simulink model "fishhook_test"  (Simulink 10.1)
settings: Solver=ode45  StartTime=0  StopTime=20  FixedStep=0.002  RelTol=1e-3  AbsTol=1e-6
PreLoadFcn:
  | m=7620;
  | a=3.105;
  | b=1.385;
  | mu=0.85;
  | g=9.8;
  | k1=-220;
  | k2=-480;
libraries: simulink x2, Solver_SF x1
settings Model: Creator=bduprey  LastModifiedBy=Lenovo  ExtModeTrigMode=oneshot  ExtModeArmWhenConnect=off
settings SolverCC: AutoScaleAbsTol=off
settings DataIOCC: SignalLoggingSaveFormat=ModelDataLogs
settings OptimizationCC: BlockReduction=off  BooleanDataType=off  ExpressionDepthLimit=2147483647
settings DebuggingCC: SaveWithParameterizedLinksMsg=none  SignalResolutionControl=TryResolveAllWithWarning  MultiTaskDSMMsg=warning  MultiTaskCondExecSysMsg=none  FcnCallInpInsideContextMsg=warning  StateNameClashWarn=warning
settings HardwareCC: TargetUnknown=on
settings RTWCC: TemplateMakefile=grt_vc.tmf
settings GRTTargetCC: TargetFcnLib=ansi_tfl_tmw.mat

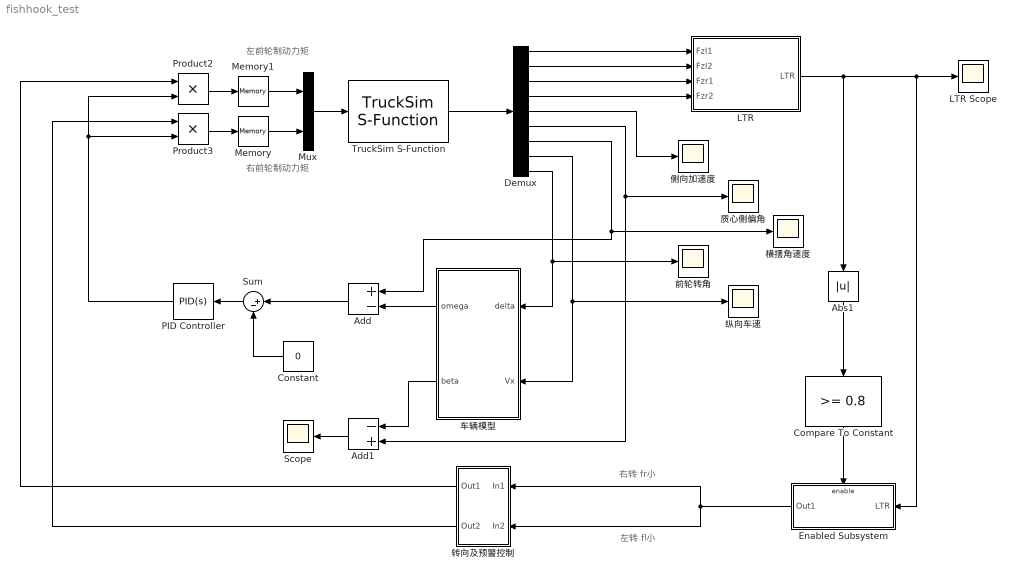
== system fishhook_test ==
  note: 左前轮制动力矩
  note: 左转 fl小
  note: 右转 fr小
  note: 右前轮制动力矩
  Abs1 : Abs
  Add : Sum  Inputs=+-
  Add1 : Sum  Inputs=-+
  Compare To Constant : simulink/Logic and Bit Operations/Compare To Constant  relop=>=  const=0.8  OutDataTypeStr=boolean
  Constant : Constant  Value=0
  Demux : Demux  Outputs=9
  Enabled Subsystem : Subsystem  TreatAsAtomicUnit=on
  LTR : Subsystem
  LTR Scope : Scope
  Memory : Memory
  Memory1 : Memory
  Mux : Mux  Inputs=2
  PID Controller : simulink/Continuous/PID Controller  Controller=PID  Form=Parallel  TimeDomain=Continuous-time  UseExternalTs=off  SampleTime=-1  IntegratorMethod=Forward Euler  FilterMethod=Forward Euler  ControllerParametersSource=internal  P=5  I=2  D=1  UseFilter=on  N=100  TunerSelectOption=Transfer Function Based (PID Tuner App)  InitialConditionSource=internal  InitialConditionForIntegrator=0  InitialConditionForFilter=0  DifferentiatorICPrevScaledInput=0  ExternalReset=none  TrackingMode=off  Kt=1  LimitOutput=off  UpperSaturationLimit=inf  LowerSaturationLimit=-inf  LinearizeAsGain=on  AntiWindupMode=none  Kb=1  POutMin=[]  POutMax=[]  IOutMin=[]  IOutMax=[]  DOutMin=[]  DOutMax=[]  NOutMin=[]  NOutMax=[]  SumOutMin=[]  SumOutMax=[]  SaturationOutMin=[]  SaturationOutMax=[]  PParamMin=[]  PParamMax=[]  IParamMin=[]  IParamMax=[]  DParamMin=[]  DParamMax=[]  NParamMin=[]  NParamMax=[]  KbParamMin=[]  KbParamMax=[]  KtParamMin=[]  KtParamMax=[]  KbOutMin=[]  KbOutMax=[]  KtOutMin=[]  KtOutMax=[]  IntegratorOutMin=[]  IntegratorOutMax=[]  FilterOutMin=[]  FilterOutMax=[]  SumI1OutMin=[]  SumI1OutMax=[]  SumI2OutMin=[]  SumI2OutMax=[]  SumI3OutMin=[]  SumI3OutMax=[]  SumI4OutMin=[]  SumI4OutMax=[]  SumDOutMin=[]  SumDOutMax=[]  DifferentiatorOutMin=[]  DifferentiatorOutMax=[]  FilterDiffOutCoefMin=[]  FilterDiffOutCoefMax=[]  ReciprocalOutMin=[]  ReciprocalOutMax=[]  SumDenOutMin=[]  SumDenOutMax=[]  SumNumOutMin=[]  SumNumOutMax=[]  DivideOutMin=[]  DivideOutMax=[]  UdiffTsProdOutMin=[]  UdiffTsProdOutMax=[]  NTsProdOutMin=[]  NTsProdOutMax=[]  UintegralTsProdOutMin=[]  UintegralTsProdOutMax=[]  UngainTsProdOutMin=[]  UngainTsProdOutMax=[]  IntegratorContinuousStateAttributes=''  IntegratorStateMustResolveToSignalObject=off  IntegratorRTWStateStorageClass=Auto  FilterContinuousStateAttributes=''  FilterStateMustResolveToSignalObject=off  FilterRTWStateStorageClass=Auto  ParallelPVariant=InternalParameters  IdealPVariant=Disabled  IVariant=InternalParameters  DVariant=InternalParameters  IntegratorVariant=Continuous  SatVariant=Disabled  AWVariant=Passthrough  PCopyVariant=Disabled  TRVariant=Disabled  FdbkBlocksVariant=Forward  IdealPFdbkVariant=Disabled  SatFdbkVariant=Disabled  DerivativeFilterVariant=ContFilter  NVariant=InternalParameters  NCopyVariant=Disabled  FilterICVariant=InternalICsFilter  IntegratorICVariant=InternalICs  ExternalResetVariant=Disabled  TRSumVariant=Passthrough  SumFdbkVariant=Disabled  SumVariant=Sum_PID  TsampFilterVariant=InternalTs  TsampNgainVariant=Passthrough  TsampIntegralVariant=Passthrough
  Product2 : Product
  Product3 : Product
  Scope : Scope
  Sum : Sum  Inputs=|+-
  TruckSim S-Function : Solver_SF/TruckSim S-Function  Priority=1  VehicleCode=i_s  SIMFILE=simfile.sim
      settings: AttributesFormatString=Vehicle Code: %<VehicleCode>
  侧向加速度 : Scope
  前轮转角 : Scope
  横摆角速度 : Scope
  纵向车速 : Scope
  质心侧偏角 : Scope
  车辆模型 : Subsystem
  转向及预警控制 : Subsystem
  wires:
  Mux/1 -> TruckSim S-Function/1
  TruckSim S-Function/1 -> Demux/1
  Demux/1 -> LTR/1(Fzl1)
  Demux/2 -> LTR/2(Fzl2)
  Demux/5 -> 侧向加速度/1
  Demux/6 -> Add1/2, 质心侧偏角/1
  Demux/7 -> Add/1, 横摆角速度/1
  LTR/1(LTR) -> Abs1/1, LTR Scope/1, Enabled Subsystem/1(LTR)
  Enabled Subsystem/1(Out1) -> 转向及预警控制/2(In2), 转向及预警控制/1(In1)
  Abs1/1 -> Compare To Constant/1
  Compare To Constant/1 -> Enabled Subsystem/Enable
  Demux/3 -> LTR/3(Fzr1)
  Demux/4 -> LTR/4(Fzr2)
  Demux/8 -> 车辆模型/2(Vx), 纵向车速/1
  Demux/9 -> 车辆模型/1(delta), 前轮转角/1
  车辆模型/1(omega) -> Add/2
  车辆模型/2(beta) -> Add1/1
  Add1/1 -> Scope/1
  Constant/1 -> Sum/2
  Add/1 -> Sum/1
  Sum/1 -> PID Controller/1
  转向及预警控制/1(Out1) -> Product2/1
  转向及预警控制/2(Out2) -> Product3/1
  Product2/1 -> Memory1/1
  Product3/1 -> Memory/1
  Memory1/1 -> Mux/1
  Memory/1 -> Mux/2
  PID Controller/1 -> Product3/2, Product2/2

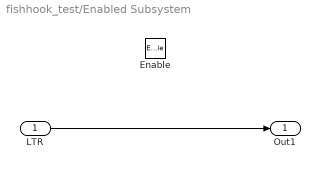
== system fishhook_test/Enabled Subsystem ==
  LTR : Inport
  Enable : EnablePort  ShowOutputPort=on
  Out1 : Outport
  wires:
  LTR/1 -> Out1/1

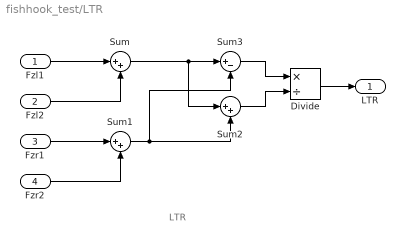
== system fishhook_test/LTR ==
  note: LTR
  Fzl1 : Inport
  Fzl2 : Inport  Port=2
  Fzr1 : Inport  Port=3
  Fzr2 : Inport  Port=4
  Divide : Product  Inputs=*/
  Sum : Sum  Inputs=|++
  Sum1 : Sum  Inputs=|++
  Sum2 : Sum  Inputs=|++
  Sum3 : Sum  Inputs=|+-
  LTR : Outport
  wires:
  Divide/1 -> LTR/1
  Sum1/1 -> Sum3/2, Sum2/2
  Fzl2/1 -> Sum/2
  Fzr1/1 -> Sum1/1
  Sum2/1 -> Divide/2
  Sum3/1 -> Divide/1
  Fzl1/1 -> Sum/1
  Fzr2/1 -> Sum1/2
  Sum/1 -> Sum2/1, Sum3/1

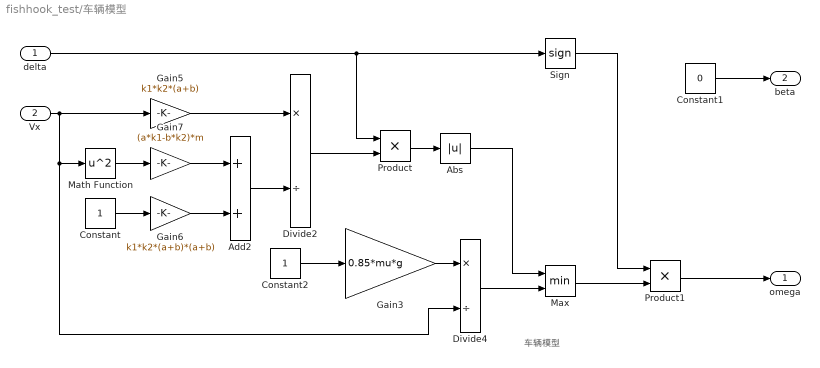
== system fishhook_test/车辆模型 ==
  note: 车辆模型
  delta : Inport
  Vx : Inport  Port=2
  Abs : Abs
  Add2 : Sum
  Constant : Constant
  Constant1 : Constant  Value=0
  Constant2 : Constant
  Divide2 : Product  Inputs=*/
  Divide4 : Product  Inputs=*/
  Gain3 : Gain  Gain=0.85*mu*g
  Gain5 : Gain  Gain=k1*k2*(a+b)
  Gain6 : Gain  Gain=k1*k2*(a+b)*(a+b)
  Gain7 : Gain  Gain=(a*k1-b*k2)*m
  Math Function : Math  Operator=square  SaturateOnIntegerOverflow=on
  Max : MinMax  Inputs=2
  Product : Product
  Product1 : Product
  Sign : Signum
  omega : Outport
  beta : Outport  Port=2
  wires:
  Vx/1 -> Gain5/1, Divide4/2, Math Function/1
  Constant/1 -> Gain6/1
  Math Function/1 -> Gain7/1
  Gain6/1 -> Add2/2
  Gain7/1 -> Add2/1
  Gain5/1 -> Divide2/1
  Add2/1 -> Divide2/2
  Constant1/1 -> beta/1
  delta/1 -> Product/1, Sign/1
  Divide2/1 -> Product/2
  Constant2/1 -> Gain3/1
  Gain3/1 -> Divide4/1
  Abs/1 -> Max/1
  Divide4/1 -> Max/2
  Max/1 -> Product1/2
  Sign/1 -> Product1/1
  Product1/1 -> omega/1
  Product/1 -> Abs/1

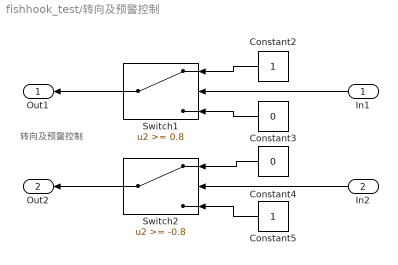
== system fishhook_test/转向及预警控制 ==
  note: 转向及预警控制
  In1 : Inport
  In2 : Inport  Port=2
  Constant2 : Constant
  Constant3 : Constant  Value=0
  Constant4 : Constant  Value=0
  Constant5 : Constant
  Switch1 : Switch  Threshold=0.8
  Switch2 : Switch  Threshold=-0.8
  Out1 : Outport
  Out2 : Outport  Port=2
  wires:
  In2/1 -> Switch2/2
  Switch2/1 -> Out2/1
  Constant3/1 -> Switch1/3
  Constant4/1 -> Switch2/1
  In1/1 -> Switch1/2
  Constant2/1 -> Switch1/1
  Switch1/1 -> Out1/1
  Constant5/1 -> Switch2/3
